simulink model "P70s"  (R2015b)
settings: Solver=VariableStepAuto  StartTime=0.0  StopTime=100  RelTol=1e-3
settings Model: Creator=xmax1946  LastModifiedBy=xmax1946

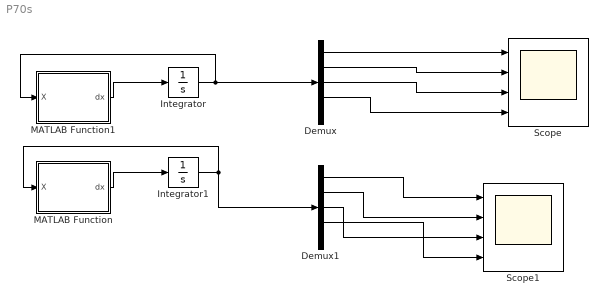
== system P70s ==
  Demux : Demux  Outputs=5
  Demux1 : Demux  Outputs=5
  Integrator : Integrator  InitialCondition=[0;0;0;0;0]
  Integrator1 : Integrator  InitialCondition=[0;0;0;0;0]
  MATLAB Function : MATLAB Function  TreatAsAtomicUnit=on
  MATLAB Function1 : MATLAB Function  TreatAsAtomicUnit=on
  Scope : Scope  NumInputPorts=4
  Scope1 : Scope  NumInputPorts=4
  wires:
  MATLAB Function1/1(dx) -> Integrator/1
  MATLAB Function/1(dx) -> Integrator1/1
  Integrator/1 -> Demux/1, MATLAB Function1/1(X)
  Integrator1/1 -> MATLAB Function/1(X), Demux1/1
  Demux/1 -> Scope/1
  Demux/2 -> Scope/2
  Demux/3 -> Scope/3
  Demux/4 -> Scope/4
  Demux1/1 -> Scope1/1
  Demux1/2 -> Scope1/2
  Demux1/3 -> Scope1/3
  Demux1/4 -> Scope1/4

== matlab function P70s/MATLAB Function1 ==
  data: dx output; X input
function dx  = fcn(X)
A=[0,-1,0,0,-4;0,0,1,0,1;0,1,0,0,2;-2,1,0,-2,4;0,0,0,0,-2];
B=[0;1;0;0;0];
u=1;
dx=A*X+B*u;

== matlab function P70s/MATLAB Function ==
  data: dx output; X input
function dx  = fcn(X)
A=[0,-1,0,0,-4;0,0,1,0,1;0,1,0,0,2;-2,1,0,-2,4;0,0,0,0,-2];
B=[0;1;0;0;0];
K=[0,8,0,17,0];
u=1-K*X;
dx=A*X+B*u;
